simulink model "motore_PI"  (R2022a)
settings: Solver=ode45  StartTime=0.0  StopTime=1  MaxStep=0.001  RelTol=1e-3
values from neighbouring files (symbols this model uses):
  d = 1 / sqrt(2)    [ex4.m]    (also in ex5.m = 1  /sqrt(2))
  KpPI = KpcPI / 4    [ex5.m]    (also in ex6.m = 0.056375)
  Ts = 0.001    [ex4.m]    (also in ex5.m; ex6.m)
  w0 = 0    [ex6.m]
undefined symbols (not defined in the file or in its folder): den, mot, num, ref
settings Model: Creator=loren  LastModifiedBy=loren
settings DataIOCC: ReturnWorkspaceOutputs=off

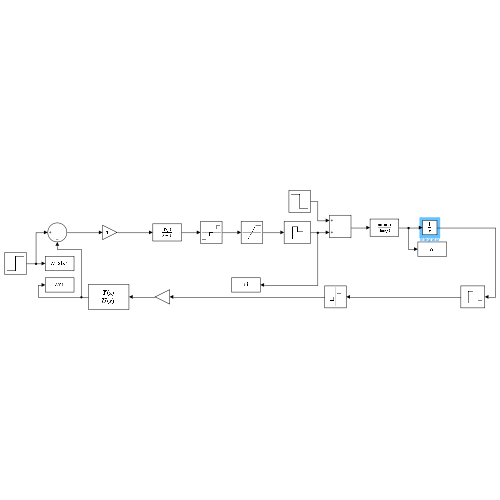
[thumbnail: Simulink's stored preview of the top-level diagram]
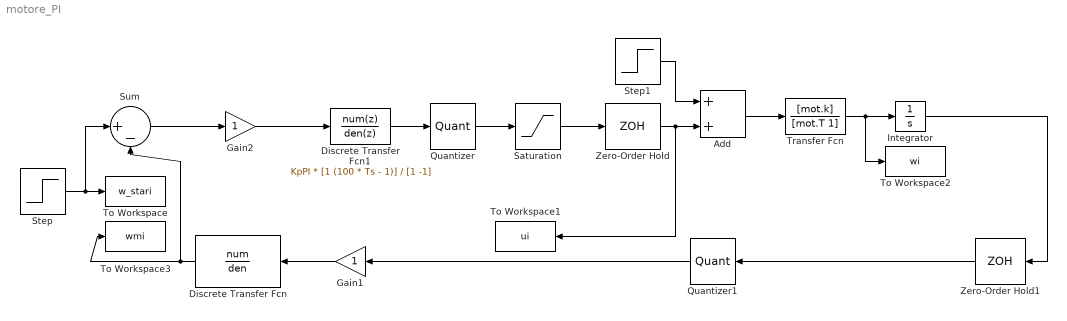
== system motore_PI ==
  Add : Sum
  Discrete Transfer Fcn : DiscreteTransferFcn  Numerator=num  Denominator=den
  Discrete Transfer Fcn1 : DiscreteTransferFcn  Numerator=KpPI * [1 (100 * Ts - 1)]  Denominator=[1 -1]
  Gain1 : Gain
  Gain2 : Gain
  Integrator : Integrator  InitialCondition=w0
  Quantizer : Quantizer  QuantizationInterval=20 / (2^16 - 1)
  Quantizer1 : Quantizer  QuantizationInterval=2 * pi / 2000
  Saturation : Saturate  UpperLimit=10  LowerLimit=-10
  Step : Step  Time=ref.t  After=ref.A  SampleTime=Ts
  Step1 : Step  Time=d.t  After=d.A  SampleTime=0
  Sum : Sum  Inputs=|+-
  To Workspace : ToWorkspace  VariableName=w_stari  SaveFormat=Timeseries  SampleTime=-1
  To Workspace1 : ToWorkspace  VariableName=ui  SaveFormat=Timeseries  SampleTime=-1
  To Workspace2 : ToWorkspace  VariableName=wi  SaveFormat=Timeseries  SampleTime=-1
  To Workspace3 : ToWorkspace  VariableName=wmi  SaveFormat=Timeseries  SampleTime=-1
  Transfer Fcn : TransferFcn  Numerator=[mot.k]  Denominator=[mot.T 1]
  Zero-Order Hold : ZeroOrderHold  SampleTime=Ts
  Zero-Order Hold1 : ZeroOrderHold  SampleTime=Ts
  wires:
  Quantizer1/1 -> Gain1/1
  Integrator/1 -> Zero-Order Hold1/1
  Sum/1 -> Gain2/1
  Discrete Transfer Fcn1/1 -> Quantizer/1
  Gain1/1 -> Discrete Transfer Fcn/1
  Quantizer/1 -> Saturation/1
  Step1/1 -> Add/1
  Saturation/1 -> Zero-Order Hold/1
  Zero-Order Hold1/1 -> Quantizer1/1
  Discrete Transfer Fcn/1 -> Sum/2, To Workspace3/1
  Add/1 -> Transfer Fcn/1
  Gain2/1 -> Discrete Transfer Fcn1/1
  Zero-Order Hold/1 -> Add/2, To Workspace1/1
  Step/1 -> To Workspace/1, Sum/1
  Transfer Fcn/1 -> Integrator/1, To Workspace2/1
